simulink model "Lab3_simulink"  (R2018a)
settings: Solver=VariableStepAuto  StartTime=0.0  StopTime=10.0  RelTol=1e-3
libraries: fl_lib x21, nesl_utility x2
settings Model: Creator=changgang  LastModifiedBy=changgang

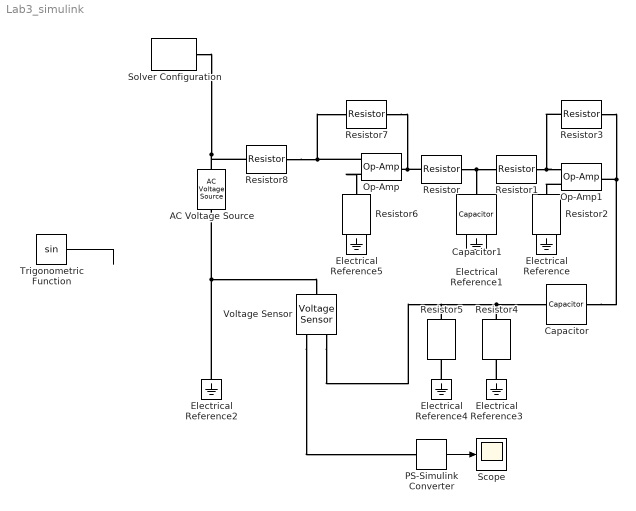
== system Lab3_simulink ==
  AC Voltage Source : fl_lib/Electrical/Electrical Sources/AC Voltage Source  amp=12 V  shift=0 deg  frequency=2 Hz  omega=0 rad/s
  Capacitor : fl_lib/Electrical/Electrical Elements/Capacitor  c=0.1 uF  r=1e-6 Ohm  g=0 1/Ohm  i_specify=off  i_priority=None  i=0 A  i_nominal_specify=off  i_nominal_unit=A  i_nominal_value=1  v_specify=off  v_priority=None  v=0 V  v_nominal_specify=off  v_nominal_unit=V  v_nominal_value=1  vc_specify=off  vc_priority=High  vc=0 V  vc_nominal_specify=off  vc_nominal_unit=V  vc_nominal_value=1
  Capacitor1 : fl_lib/Electrical/Electrical Elements/Capacitor  c=0.1 uF  r=1e-6 Ohm  g=0 1/Ohm  i_specify=off  i_priority=None  i=0 A  i_nominal_specify=off  i_nominal_unit=A  i_nominal_value=1  v_specify=off  v_priority=None  v=0 V  v_nominal_specify=off  v_nominal_unit=V  v_nominal_value=1  vc_specify=off  vc_priority=High  vc=0 V  vc_nominal_specify=off  vc_nominal_unit=V  vc_nominal_value=1
  Electrical Reference{,1..5} (6 alike) : fl_lib/Electrical/Electrical Elements/Electrical Reference
  Op-Amp : fl_lib/Electrical/Electrical Elements/Op-Amp  outI_specify=off  outI_priority=None  outI=0 A  outI_nominal_specify=off  outI_nominal_unit=A  outI_nominal_value=1
  Op-Amp1 : fl_lib/Electrical/Electrical Elements/Op-Amp  outI_specify=off  outI_priority=None  outI=0 A  outI_nominal_specify=off  outI_nominal_unit=A  outI_nominal_value=1
  PS-Simulink Converter : nesl_utility/PS-Simulink Converter  PhysicalDomain=network_engine_domain  SubClassName=ps_output  LeftPortType=input  RightPortType=output  PseudoPeriodic=off  Frequencies=[]  Unit=1  AffineConversion=off
  Resistor{,1..8} (9 alike) : fl_lib/Electrical/Electrical Elements/Resistor  R=3.3 kOhm  i_specify=off  i_priority=None  i=0 A  i_nominal_specify=off  i_nominal_unit=A  i_nominal_value=1  v_specify=off  v_priority=None  v=0 V  v_nominal_specify=off  v_nominal_unit=V  v_nominal_value=1
  Scope : Scope
  Solver Configuration : nesl_utility/Solver Configuration  PhysicalDomain=network_engine_domain  SubClassName=solver  LeftPortType=input  RightPortType=generic  Tones=[]  Harmonics=[]  SimulateNoise=off  Profile=off  UseLocalSampling=off  EnableSwitchedLinearOptims=on  FrequencyDomain=off  UseCCode=off  RelTol=0.001  AbsTol=1e-06  MinStep=1e-09  ToWorkspace=off  RevertToSquareIcSolve=off  NumHomotopyIterations=100  PhasorMode=off  PhasorModeNumHarmonics=1  DoDC=off  ResidualTolerance=1e-09  UseLocalSolver=off  LocalSolverChoice=NE_BACKWARD_EULER_ADVANCER  LocalSolverSampleTime=0.001  DoFixedCost=off  MaxNonlinIter=3  MaxModeIter=2  LinearAlgebra=Sparse  EquationFormulation=NE_TIME_EF  DelaysMemoryBudget=1024  AutomaticFiltering=on  FilteringTimeConstant=0.001
  Trigonometric Function : Trigonometry
  Voltage Sensor : fl_lib/Electrical/Electrical Sensors/Voltage Sensor
  wires:
  PS-Simulink Converter/1 -> Scope/1
  Trigonometric Function/1 -> ?
  connections:
  Resistor/LConn1 -- Resistor7/RConn1 -- Op-Amp/RConn1
  Resistor/RConn1 -- Capacitor1/LConn1 -- Resistor1/LConn1
  Resistor1/RConn1 -- Resistor3/LConn1 -- Op-Amp1/LConn1
  Electrical Reference1/LConn1 -- Capacitor1/RConn1
  Op-Amp1/LConn2 -- Resistor2/LConn1
  Electrical Reference/LConn1 -- Resistor2/RConn1
  Resistor3/RConn1 -- Op-Amp1/RConn1 -- Capacitor/RConn1
  Electrical Reference2/LConn1 -- Voltage Sensor/LConn1 -- AC Voltage Source/RConn1
  Op-Amp/LConn2 -- Resistor6/LConn1
  Electrical Reference5/LConn1 -- Resistor6/RConn1
  Op-Amp/LConn1 -- Resistor8/RConn1 -- Resistor7/LConn1
  Voltage Sensor/RConn1 -- PS-Simulink Converter/LConn1
  Electrical Reference3/LConn1 -- Resistor4/RConn1
  Resistor4/LConn1 -- Voltage Sensor/RConn2 -- Resistor5/LConn1 -- Capacitor/LConn1
  Electrical Reference4/LConn1 -- Resistor5/RConn1
  Resistor8/LConn1 -- AC Voltage Source/LConn1 -- Solver Configuration/RConn1
